simulink model "Zbiorniki_lqr"  (R2015a)
settings: Solver=ode5  SolverMode=SingleTasking  StartTime=0.0  StopTime=999  FixedStep=T0  RelTol=1e-3  AbsTol=1e-6
values from neighbouring files (symbols this model uses):
  K = lqr(A,B,Q,r)    [regulator_LQR.m]
undefined symbols (not defined in the file or in its folder): h1, h2, h3
undefined symbols (not defined in the file): RTDAC4PCIBaseAddress, T0
libraries: simulink x3
settings Model: SimulationMode=external  ExtModeTrigDuration=300000  Creator=jims  LastModifiedBy=Student
settings DataIOCC: ExternalInput=[]  InitialState=[]  LimitDataPoints=off  MaxDataPoints=5000  SignalLoggingSaveFormat=ModelDataLogs  SaveOutput=off  SaveTime=off  SignalLoggingName=sigsOut
settings OptimizationCC: BooleanDataType=off  ExpressionDepthLimit=2147483647  InitFltsAndDblsToZero=on
settings DebuggingCC: SaveWithParameterizedLinksMsg=none  UnderspecifiedInitializationDetection=Classic  MergeDetectMultiDrivingBlocksExec=none  SignalResolutionControl=TryResolveAllWithWarning  MultiTaskDSMMsg=warning  MultiTaskCondExecSysMsg=none  IntegerOverflowMsg=none  FcnCallInpInsideContextMsg=UseLocalSettings  StateNameClashWarn=warning  IntegerSaturationMsg=none
settings HardwareCC: TargetLongLongMode=on  TargetEndianess=LittleEndian  TargetHWDeviceType=MATLAB Host  ProdEqTarget=off
settings RTWCC: SystemTargetFile=rtwin.tlc  TemplateMakefile=RTDAC_win.tmf  Description=Real-Time Windows Target
settings TargetCC: ModelReferenceCompliant=off  CompOptLevelCompliant=off

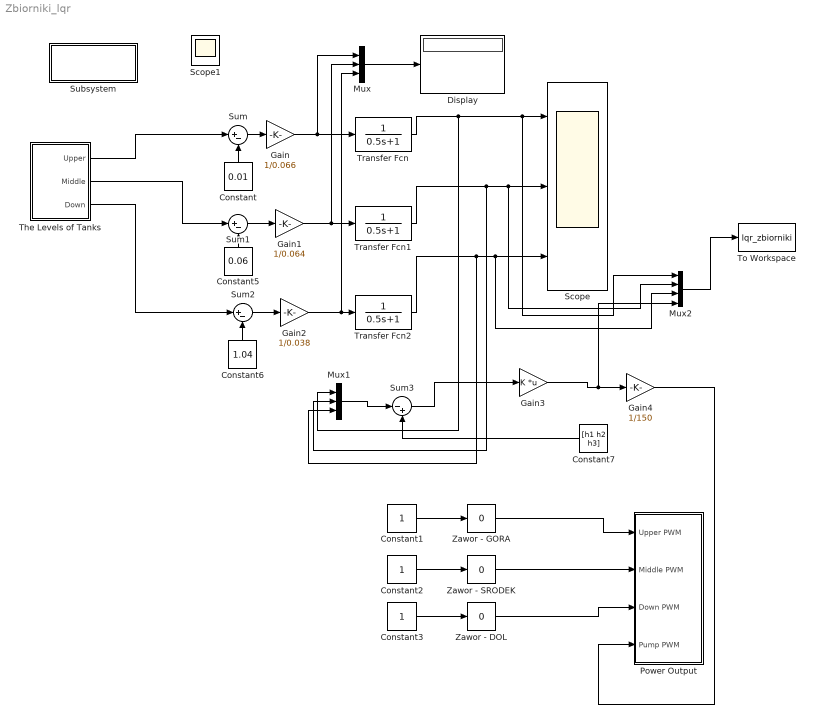
== system Zbiorniki_lqr ==
  Constant : Constant  Value=0.01
  Constant1 : Constant
  Constant2 : Constant
  Constant3 : Constant
  Constant5 : Constant  Value=0.06
  Constant6 : Constant  Value=1.04
  Constant7 : Constant  Value=[h1 h2 h3]
  Display : Display
  Gain : Gain  Gain=1/0.066
  Gain1 : Gain  Gain=1/0.064
  Gain2 : Gain  Gain=1/0.038
  Gain3 : Gain  Gain=K  Multiplication=Matrix(K*u)
  Gain4 : Gain  Gain=1/150
  Mux : Mux  Inputs=3
  Mux1 : Mux  Inputs=3
  Mux2 : Mux
  Power Output : Subsystem
  Scope : Scope  NumInputPorts=3
      settings: TimeRange=120  YMin=0.65~0.55~0  YMax=0.95~0.775~25  SaveName=Lev  MaxDataPoints=20000
  Subsystem : Subsystem
      settings: OpenFcn=T0=0.01
      mask Display: disp('Wczytaj T0')
  Sum : Sum  Inputs=|+-
  Sum1 : Sum  Inputs=|+-
  Sum2 : Sum  Inputs=|+-
  Sum3 : Sum  Inputs=|-+
  The Levels of Tanks : Subsystem
  To Workspace : ToWorkspace  VariableName=lqr_zbiorniki  SaveFormat=Structure With Time  SampleTime=-1
  Transfer Fcn : TransferFcn  Denominator=[0.5 1]
  Transfer Fcn1 : TransferFcn  Denominator=[0.5 1]
  Transfer Fcn2 : TransferFcn  Denominator=[0.5 1]
  Zawor - DOL : simulink/Math Operations/Slider Gain  low=0  gain=0  high=1
  Zawor - GORA : simulink/Math Operations/Slider Gain  low=0  gain=0  high=1
  Zawor - SRODEK : simulink/Math Operations/Slider Gain  low=0  gain=0  high=1
  Scope1 : Scope
      settings: YMin=-500  YMax=6500
  wires:
  Mux/1 -> Display/1
  Constant2/1 -> Zawor - SRODEK/1
  Constant3/1 -> Zawor - DOL/1
  Zawor - SRODEK/1 -> Power Output/2(Middle PWM)
  Gain4/1 -> Power Output/4(Pump PWM)
  Constant1/1 -> Zawor - GORA/1
  Zawor - DOL/1 -> Power Output/3(Down PWM)
  Zawor - GORA/1 -> Power Output/1(Upper PWM)
  The Levels of Tanks/1(Upper) -> Sum/1
  The Levels of Tanks/2(Middle) -> Sum1/1
  The Levels of Tanks/3(Down) -> Sum2/1
  Constant/1 -> Sum/2
  Constant5/1 -> Sum1/2
  Constant6/1 -> Sum2/2
  Sum/1 -> Gain/1
  Sum1/1 -> Gain1/1
  Sum2/1 -> Gain2/1
  Gain/1 -> Mux/1, Transfer Fcn/1
  Gain1/1 -> Mux/2, Transfer Fcn1/1
  Gain2/1 -> Mux/3, Transfer Fcn2/1
  Transfer Fcn/1 -> Mux1/1, Mux2/1, Scope/1
  Transfer Fcn1/1 -> Mux1/2, Mux2/2, Scope/2
  Transfer Fcn2/1 -> Mux1/3, Mux2/3, Scope/3
  Constant7/1 -> Sum3/2
  Mux1/1 -> Sum3/1
  Sum3/1 -> Gain3/1
  Gain3/1 -> Mux2/4, Gain4/1
  Mux2/1 -> To Workspace/1

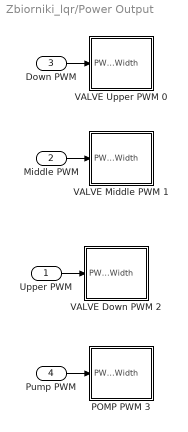
== system Zbiorniki_lqr/Power Output ==
  Upper PWM : Inport
  Middle PWM : Inport  Port=2
  Down PWM : Inport  Port=3
  Pump PWM : Inport  Port=4
  POMP PWM 3 : Subsystem  mask(PWM Module){BaseAddress=RTDAC4PCIBaseAddress, ChanIdx=3, ChanMode=12 Bit, ChanPresc=30, SetOutputsFlag=on, SetOutputsValue=0, T0=T0}
      mask prompts: BaseAddress "IO Base Address:"; ChanIdx "Channel:"; ChanMode "Channel Mode:"; ChanPresc "Channel Prescaler:"; SetOutputsFlag "Set Outputs At Termination"; SetOutputsValue "Termination Outputs:"; T0 "Sample Time (sec):"
      mask help: RT-DAC PCI Device Driver
      mask Help: Set up each field for your specific hardware configuration.
      mask TypeOptions ChanIdx: 0 | 1 | 2 | 3
      mask TypeOptions ChanMode: 8 Bit | 12 Bit
      mask Display: plot(0,0,100,100,[90,80,80,11,11],[90,90,20,20,80],[11,80],[80,80],[80,80],[20,14],[80,85,85,80],[45,45,66,66],[45,45,74,74],[20,13,13,20],[15,27,27,15,15],[75,75,26,26,75],[33,48,48,33,33],[75,75,55,55,75],[55,55,71,71,55],[55,75,75,55,55],[33,41,41,33,33],[50,50,27,27,50],[48,56,56,48,48],[50,50,27,27,50],[62,70,70,62,62],[50,50,27,27,50])
  VALVE Down PWM 2 : Subsystem  mask(PWM Module){BaseAddress=RTDAC4PCIBaseAddress, ChanIdx=2, ChanMode=12 Bit, ChanPresc=30, SetOutputsFlag=on, SetOutputsValue=0, T0=T0}
      mask prompts: BaseAddress "IO Base Address:"; ChanIdx "Channel:"; ChanMode "Channel Mode:"; ChanPresc "Channel Prescaler:"; SetOutputsFlag "Set Outputs At Termination"; SetOutputsValue "Termination Outputs:"; T0 "Sample Time (sec):"
      mask help: RT-DAC PCI Device Driver
      mask Help: Set up each field for your specific hardware configuration.
      mask TypeOptions ChanIdx: 0 | 1 | 2 | 3
      mask TypeOptions ChanMode: 8 Bit | 12 Bit
      mask Display: plot(0,0,100,100,[90,80,80,11,11],[90,90,20,20,80],[11,80],[80,80],[80,80],[20,14],[80,85,85,80],[45,45,66,66],[45,45,74,74],[20,13,13,20],[15,27,27,15,15],[75,75,26,26,75],[33,48,48,33,33],[75,75,55,55,75],[55,55,71,71,55],[55,75,75,55,55],[33,41,41,33,33],[50,50,27,27,50],[48,56,56,48,48],[50,50,27,27,50],[62,70,70,62,62],[50,50,27,27,50])
  VALVE Middle PWM 1 : Subsystem  mask(PWM Module){BaseAddress=RTDAC4PCIBaseAddress, ChanIdx=1, ChanMode=12 Bit, ChanPresc=30, SetOutputsFlag=on, SetOutputsValue=0, T0=T0}
      mask prompts: BaseAddress "IO Base Address:"; ChanIdx "Channel:"; ChanMode "Channel Mode:"; ChanPresc "Channel Prescaler:"; SetOutputsFlag "Set Outputs At Termination"; SetOutputsValue "Termination Outputs:"; T0 "Sample Time (sec):"
      mask help: RT-DAC PCI Device Driver
      mask Help: Set up each field for your specific hardware configuration.
      mask TypeOptions ChanIdx: 0 | 1 | 2 | 3
      mask TypeOptions ChanMode: 8 Bit | 12 Bit
      mask Display: plot(0,0,100,100,[90,80,80,11,11],[90,90,20,20,80],[11,80],[80,80],[80,80],[20,14],[80,85,85,80],[45,45,66,66],[45,45,74,74],[20,13,13,20],[15,27,27,15,15],[75,75,26,26,75],[33,48,48,33,33],[75,75,55,55,75],[55,55,71,71,55],[55,75,75,55,55],[33,41,41,33,33],[50,50,27,27,50],[48,56,56,48,48],[50,50,27,27,50],[62,70,70,62,62],[50,50,27,27,50])
  VALVE Upper PWM 0 : Subsystem  mask(PWM Module){BaseAddress=RTDAC4PCIBaseAddress, ChanIdx=0, ChanMode=12 Bit, ChanPresc=30, SetOutputsFlag=on, SetOutputsValue=0, T0=T0}
      mask prompts: BaseAddress "IO Base Address:"; ChanIdx "Channel:"; ChanMode "Channel Mode:"; ChanPresc "Channel Prescaler:"; SetOutputsFlag "Set Outputs At Termination"; SetOutputsValue "Termination Outputs:"; T0 "Sample Time (sec):"
      mask help: RT-DAC PCI Device Driver
      mask Help: Set up each field for your specific hardware configuration.
      mask TypeOptions ChanIdx: 0 | 1 | 2 | 3
      mask TypeOptions ChanMode: 8 Bit | 12 Bit
      mask Display: plot(0,0,100,100,[90,80,80,11,11],[90,90,20,20,80],[11,80],[80,80],[80,80],[20,14],[80,85,85,80],[45,45,66,66],[45,45,74,74],[20,13,13,20],[15,27,27,15,15],[75,75,26,26,75],[33,48,48,33,33],[75,75,55,55,75],[55,55,71,71,55],[55,75,75,55,55],[33,41,41,33,33],[50,50,27,27,50],[48,56,56,48,48],[50,50,27,27,50],[62,70,70,62,62],[50,50,27,27,50])
  wires:
  Down PWM/1 -> VALVE Upper PWM 0/1(PWM Width)
  Middle PWM/1 -> VALVE Middle PWM 1/1(PWM Width)
  Upper PWM/1 -> VALVE Down PWM 2/1(PWM Width)
  Pump PWM/1 -> POMP PWM 3/1(PWM Width)

== system Zbiorniki_lqr/Subsystem ==

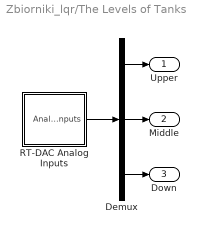
== system Zbiorniki_lqr/The Levels of Tanks ==
  Demux : Demux  Outputs=3
  RT-DAC Analog Inputs : Subsystem  mask(Analog Input Module){BaseAddress=RTDAC4PCIBaseAddress, Chan=[0 1 2], Gain=[1 1 1], T0=0.05}
      mask prompts: BaseAddress "Base Address:"; Chan "Channel:"; T0 "Sample Time (sec):"
      mask help: RT-DAC PCI Device Driver
      mask Help: Set up each field for your specific hardware configuration.
      mask Display: plot(0,0,100,100,[90,80,80,11,11],[90,90,20,20,80],[11,80],[80,80],[80,80],[20,14],[80,85,85,80],[45,45,66,66],[45,45,74,74],[20,13,13,20],[15,27,27,15,15],[75,75,26,26,75],[33,48,48,33,33],[75,75,55,55,75],[55,55,71,71,55],[55,75,75,55,55],[33,41,41,33,33],[50,50,27,27,50],[48,56,56,48,48],[50,50,27,27,50],[62,70,70,62,62],[50,50,27,27,50])
  Upper : Outport
  Middle : Outport  Port=2
  Down : Outport  Port=3
  wires:
  RT-DAC Analog Inputs/1(Analog Inputs) -> Demux/1
  Demux/1 -> Upper/1
  Demux/2 -> Middle/1
  Demux/3 -> Down/1

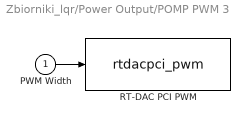
== system Zbiorniki_lqr/Power Output/POMP PWM 3 ==
  PWM Width : Inport
  "RT-DAC PCI PWM " : S-Function  FunctionName=rtdacpci_pwm  Parameters=BaseAddress, ChanIdx, ChanMode, ChanPresc, SetOutputsFlag, SetOutputsValue, T0
  wires:
  PWM Width/1 -> "RT-DAC PCI PWM "/1

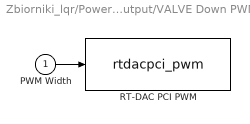
== system Zbiorniki_lqr/Power Output/VALVE Down PWM 2 ==
  PWM Width : Inport
  "RT-DAC PCI PWM " : S-Function  FunctionName=rtdacpci_pwm  Parameters=BaseAddress, ChanIdx, ChanMode, ChanPresc, SetOutputsFlag, SetOutputsValue, T0
  wires:
  PWM Width/1 -> "RT-DAC PCI PWM "/1

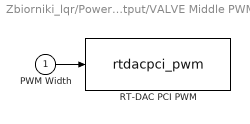
== system Zbiorniki_lqr/Power Output/VALVE Middle PWM 1 ==
  PWM Width : Inport
  "RT-DAC PCI PWM " : S-Function  FunctionName=rtdacpci_pwm  Parameters=BaseAddress, ChanIdx, ChanMode, ChanPresc, SetOutputsFlag, SetOutputsValue, T0
  wires:
  PWM Width/1 -> "RT-DAC PCI PWM "/1

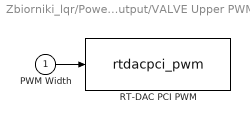
== system Zbiorniki_lqr/Power Output/VALVE Upper PWM 0 ==
  PWM Width : Inport
  "RT-DAC PCI PWM " : S-Function  FunctionName=rtdacpci_pwm  Parameters=BaseAddress, ChanIdx, ChanMode, ChanPresc, SetOutputsFlag, SetOutputsValue, T0
  wires:
  PWM Width/1 -> "RT-DAC PCI PWM "/1

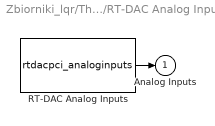
== system Zbiorniki_lqr/The Levels of Tanks/RT-DAC Analog Inputs ==
  RT-DAC Analog Inputs : S-Function  FunctionName=rtdacpci_analoginputs  Parameters=BaseAddress, Chan, Gain, T0
  Analog Inputs : Outport
  wires:
  RT-DAC Analog Inputs/1 -> Analog Inputs/1
